simulink model "carPlant_smoothUp_followerStopper_10"  (R2018b)
settings: Solver=VariableStepAuto  StartTime=0.0  StopTime=inf  RelTol=1e-3
undefined symbols (not defined in the file or in its folder): Angular, Linear
libraries: robotlib x13, autolibshared x10, vehdynlibsteering x10
(part 1 of 2)
settings Model: Creator=ckreienk  LastModifiedBy=ckreienk

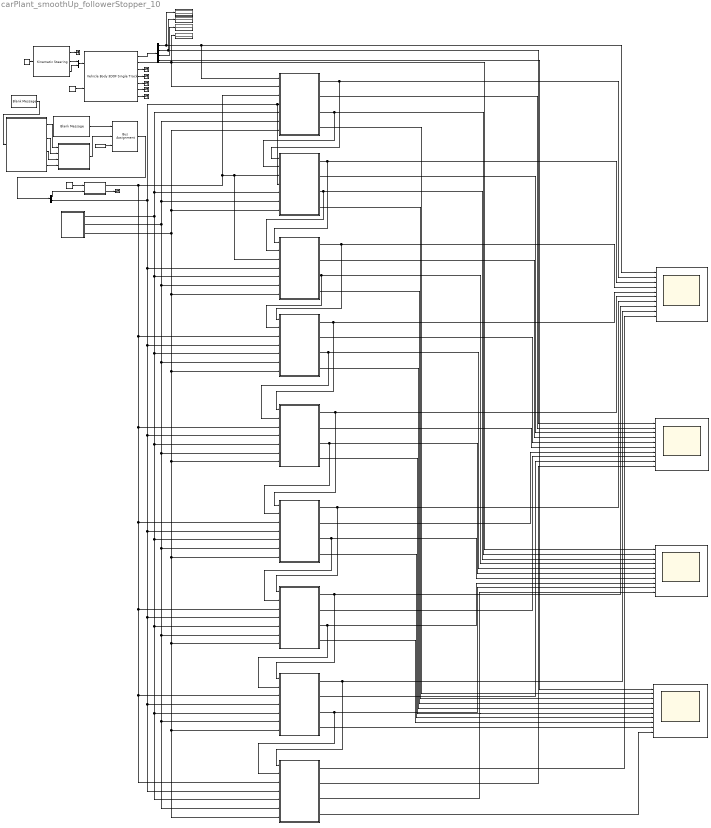
== system carPlant_smoothUp_followerStopper_10 ==
  Acceleration : Scope  NumInputPorts=10
  Blank Message : robotlib/Blank Message  messageClass=Message  entityType=geometry_msgs/Point  messageType=geometry_msgs/Point  SampleTime=inf
      settings: SourceProductBaseCode=RO
  Blank Message Leader : robotlib/Blank Message  messageClass=Message  entityType=geometry_msgs/Twist  messageType=geometry_msgs/Twist  SampleTime=inf
      settings: SourceProductBaseCode=RO
  Bus Assignment7 : BusAssignment  AssignedSignals=Linear.X,Angular.Z
  Bus Selector : BusSelector  OutputSignals=Linear.X,Angular.Z
  Bus Selector2 : BusSelector  OutputSignals=InertFrm.Geom.Disp.X,InertFrm.Geom.Disp.Y,InertFrm.Geom.Disp.Z,BdyFrm.Cg.Acc.xddot
  Constant12 : Constant
  Constant3 : Constant  Value=0
  Dead Man's Switch : Subsystem  TreatAsAtomicUnit=on  mask{stepSize=0.05, timeout=0.2}
      mask prompts: stepSize "Simulation step size"; timeout "Timeout (in seconds)"
      mask help: Interprets whether a new message has been recently received, and if so permits the data in 'value' to be passed through. Otherwise, 0 is outputted from 'safeValue'
      mask Help: Interprets whether a new message has been recently received, and if so permits the data in 'value' to be passed through. Otherwise, 0 is outputted from 'safeValue'
  Display{1..3,7} (4 alike) : Display
  Follower 1 : Subsystem
  Follower 2 : Subsystem
  Follower 3 : Subsystem
  Follower 4 : Subsystem
  Follower 5 : Subsystem
  Follower 6 : Subsystem
  Follower 7 : Subsystem
  Follower 8 : Subsystem
  Follower 9 : Subsystem
  Kinematic Steering : vehdynlibsteering/Kinematic Steering  StrgType=Rack and pinion  StrgRatioType=Constant  Loc=Front  NrmlFctr=0.01  TrckWdth=1  WhlBase=1.524  Db=0  StrgRng=1.25*pi  StrgAngBpts="[-6.2832   -5.0265   -3.7699   -2.5133   -1.2566         0    1.2566    2.5133    3.7699    5.0265    6.2832]"  StrgRatioTbl=|  StrgRatio=100  StrgArmLngth=0.1  RckCsLngth=0.5  TieRodLngth=0.248  D=0.2  PnnRadius=0.0057  PnnRadiusTbl="[0.0055    0.0055    0.0056    0.0057    0.0058    0.0057    0.0057    0.0057    0.0056    0.0055    0.0055]"  RodLngth=0.1  ParaArmLngth=0.9  aMode=2
      | [13.5000   13.3750   13.2500   13.1250   13.0000   13.0000   13.0000   13.1250   13.2500   13.3750   13.5000
      | ]
      settings: SourceProductName=Vehicle Dynamics Blockset
  Lead Vehicle : autolibshared/Vehicle Body 3DOF Single Track  trackMode=Dual  inputMode=External longitudinal velocity  frontSteerMode=on  rearSteerMode=off  windMode=off  muMode=off  extFMode=off  extMMode=off  aMode=2  NF=2  NR=2  m=2000  a=1.4  b=1.6  h=0.35  X_o=45  xdot_o=0  CalphaMode=off  sigmaMode=on  d=0  w=[1.4,1.4]  Cy_f=12e3  Cy_r=11e3  sigma_f=.1  sigma_r=.1  alpha_f_brk=[-.1 .1]  Cy_f_data=[-9e3 9e3]  alpha_r_brk=[-.1 .1]  Cy_r_data=[-9e3 9e3]  Y_o=0  ydot_o=0  Izz=4000  psi_o=0  r_o=0  Af=2  Cd=.3  Cl=.1  Cpm=.1  beta_w=[0:0.01:0.3]  Cs=[0:0.03:0.9]  Cym=[0:0.01:0.3]  Pabs=101325  Tair=273  g=9.81  mu=1  xdot_tol=.01  Fznom=5000  Fxtire_sat=7e4  Fytire_sat=7e4  longOff=0  latOff=0  vertOff=0
      settings: SourceProductName=Powertrain Blockset  SourceProductBaseCode=PW
  MATLAB Function : MATLAB Function  TreatAsAtomicUnit=on
  Parameters : Subsystem
  Random Number : RandomNumber  Mean=3  Variance=3  SampleTime=0.1
  Steering angle : Constant  Value=0.0
  Terminator{5..10,15} (7 alike) : Terminator
  Vector Concatenate : Concatenate
  Velocity : Scope  NumInputPorts=10
  X-Position : Scope  NumInputPorts=10
  Y-Position : Scope  NumInputPorts=10
  smoothUp Parameters : Subsystem
  wires:
  Lead Vehicle/6 -> Terminator9/1
  Bus Selector2/3 -> Display3/1  "<Z>"
  smoothUp Parameters/1(max_speed) -> MATLAB Function/1(max_speed)
  Bus Selector/1 -> Dead Man's Switch/2(value)  "<X>"
  Blank Message Leader/1 -> Bus Assignment7/1
  MATLAB Function/1(u_out) -> Bus Assignment7/2
  Bus Selector2/4 -> Acceleration/1  "<xddot>"
  Lead Vehicle/4 -> Terminator7/1
  Lead Vehicle/2 -> Display7/1, Velocity/1, Follower 1/2(V_(n-1))
  Lead Vehicle/3 -> Terminator6/1
  Lead Vehicle/1 -> Bus Selector2/1
  Dead Man's Switch/2(timedOut) -> Terminator15/1
  Blank Message/1 -> smoothUp Parameters/1(In1)
  Bus Selector2/2 -> Y-Position/1, Display2/1  "<Y>"
  Constant3/1 -> Kinematic Steering/1
  Lead Vehicle/7 -> Terminator10/1
  Kinematic Steering/3 -> Vector Concatenate/2
  Bus Selector2/1 -> Display1/1, X-Position/1, Follower 1/1(X_(n-1))  "<X>"
  Lead Vehicle/5 -> Terminator8/1
  Bus Assignment7/1 -> Bus Selector/1
  Kinematic Steering/1 -> Terminator5/1
  Kinematic Steering/2 -> Vector Concatenate/1
  Random Number/1 -> Lead Vehicle/2
  Constant12/1 -> Dead Man's Switch/1(IsNew)
  Steering angle/1 -> Bus Assignment7/3
  Vector Concatenate/1 -> Lead Vehicle/1
  Dead Man's Switch/1(safeValue) -> Follower 9/3(reference velocity), Follower 8/3(reference velocity), Follower 7/3(reference velocity), Follower 6/3(reference velocity), Follower 5/3(reference velocity), Follower 4/3(reference velocity), Follower 3/3(reference velocity), Follower 2/3(reference velocity), Follower 1/3(reference velocity)
  Bus Selector/2 -> Follower 9/4(reference angle), Follower 8/4(reference angle), Follower 7/4(reference angle), Follower 6/4(reference angle), Follower 5/4(reference angle), Follower 4/4(reference angle), Follower 3/4(reference angle), Follower 2/4(reference angle), Follower 1/4(reference angle)  "<Z>"
  Parameters/1(alpha) -> Follower 9/5(alpha), Follower 8/5(alpha), Follower 7/5(alpha), Follower 6/5(alpha), Follower 5/5(alpha), Follower 4/5(alpha), Follower 3/5(alpha), Follower 2/5(alpha), Follower 1/5(alpha)
  Parameters/2(omega_1) -> Follower 9/6(omega1), Follower 8/6(omega1), Follower 7/6(omega1), Follower 6/6(omega1), Follower 5/6(omega1), Follower 4/6(omega1), Follower 3/6(omega1), Follower 2/6(omega1), Follower 1/6(omega1)
  Parameters/3(omega_3) -> Follower 9/7(omega3), Follower 8/7(omega3), Follower 7/7(omega3), Follower 6/7(omega3), Follower 5/7(omega3), Follower 4/7(omega3), Follower 3/7(omega3), Follower 2/7(omega3), Follower 1/7(omega3)
  Follower 1/1(X_n) -> Follower 2/1(X_(n-1)), X-Position/2
  Follower 1/2(Y_n) -> Y-Position/2
  Follower 1/3(V_n) -> Follower 2/2(V_(n-1)), Velocity/2
  Follower 1/4(A_n) -> Acceleration/2
  Follower 2/1(X_n) -> Follower 3/1(X_(n-1)), X-Position/3
  Follower 2/3(V_n) -> Follower 3/2(V_(n-1)), Velocity/3
  Follower 3/1(X_n) -> Follower 4/1(X_(n-1)), X-Position/4
  Follower 3/3(V_n) -> Follower 4/2(V_(n-1)), Velocity/4
  Follower 4/1(X_n) -> X-Position/5, Follower 5/1(X_(n-1))
  Follower 4/3(V_n) -> Follower 5/2(V_(n-1)), Velocity/5
  Follower 5/3(V_n) -> Follower 6/2(V_(n-1)), Velocity/6
  Follower 5/1(X_n) -> X-Position/6, Follower 6/1(X_(n-1))
  Follower 6/1(X_n) -> X-Position/7, Follower 7/1(X_(n-1))
  Follower 6/3(V_n) -> Follower 7/2(V_(n-1)), Velocity/7
  Follower 7/1(X_n) -> X-Position/8, Follower 8/1(X_(n-1))
  Follower 7/3(V_n) -> Velocity/8, Follower 8/2(V_(n-1))
  Follower 8/1(X_n) -> X-Position/9, Follower 9/1(X_(n-1))
  Follower 8/3(V_n) -> Velocity/9, Follower 9/2(V_(n-1))
  Follower 9/1(X_n) -> X-Position/10
  Follower 2/2(Y_n) -> Y-Position/3
  Follower 3/2(Y_n) -> Y-Position/4
  Follower 4/2(Y_n) -> Y-Position/5
  Follower 5/2(Y_n) -> Y-Position/6
  Follower 6/2(Y_n) -> Y-Position/7
  Follower 7/2(Y_n) -> Y-Position/8
  Follower 8/2(Y_n) -> Y-Position/9
  Follower 9/2(Y_n) -> Y-Position/10
  Follower 9/3(V_n) -> Velocity/10
  Follower 2/4(A_n) -> Acceleration/3
  Follower 3/4(A_n) -> Acceleration/4
  Follower 4/4(A_n) -> Acceleration/5
  Follower 5/4(A_n) -> Acceleration/6
  Follower 6/4(A_n) -> Acceleration/7
  Follower 7/4(A_n) -> Acceleration/8
  Follower 8/4(A_n) -> Acceleration/9
  Follower 9/4(A_n) -> Acceleration/10
  smoothUp Parameters/2(reference_vel) -> MATLAB Function/2(vel)
  smoothUp Parameters/3(max_accel) -> MATLAB Function/3(max_accel)
  smoothUp Parameters/4(max_decel) -> MATLAB Function/4(max_decel)

== system carPlant_smoothUp_followerStopper_10/Dead Man's Switch ==
  note: The timeout value, and step size, are critical to set correctly here.
  IsNew : Inport
  value : Inport  Port=2
  Simulate step size : Constant  Value=stepSize
  Timeout in seconds : Constant  Value=timeout
  timeout set to 0 output : MATLAB Function  TreatAsAtomicUnit=on
  safeValue : Outport  InitialOutput=[0]
  timedOut : Outport  Port=2  InitialOutput=[0]
  wires:
  Simulate step size/1 -> timeout set to 0 output/4(stepSize)
  timeout set to 0 output/2(timedOut) -> timedOut/1
  Timeout in seconds/1 -> timeout set to 0 output/3(timeout)
  value/1 -> timeout set to 0 output/2(value)
  timeout set to 0 output/1(safeValue) -> safeValue/1
  IsNew/1 -> timeout set to 0 output/1(isNew)

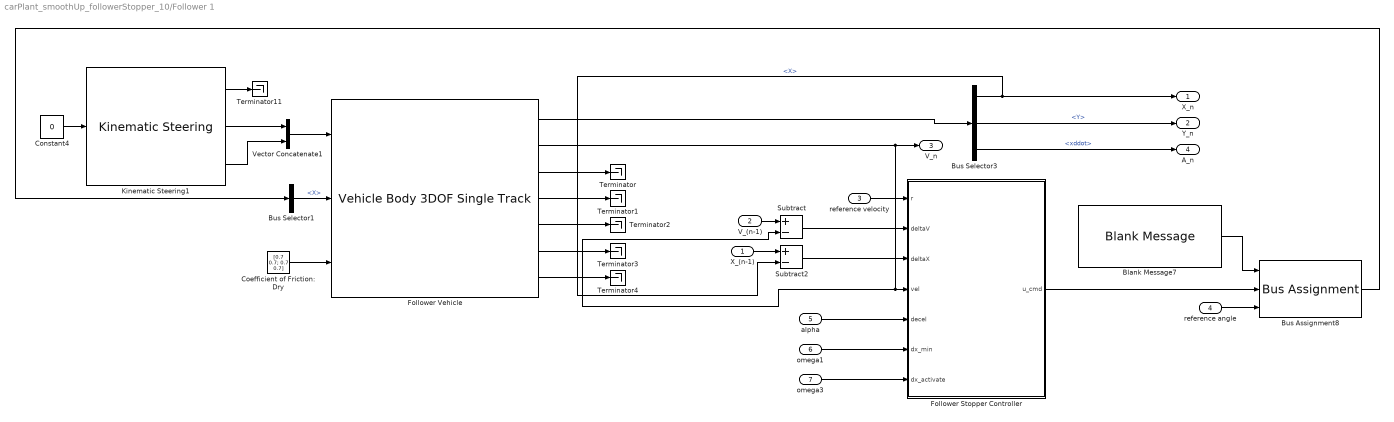
== system carPlant_smoothUp_followerStopper_10/Follower 1 ==
  X_(n-1) : Inport
  V_(n-1) : Inport  Port=2
  reference velocity : Inport  Port=3
  reference angle : Inport  Port=4
  alpha : Inport  Port=5
  omega1 : Inport  Port=6
  omega3 : Inport  Port=7
  Blank Message7 : robotlib/Blank Message  messageClass=Message  entityType=geometry_msgs/Twist  messageType=geometry_msgs/Twist  SampleTime=inf
      settings: SourceProductBaseCode=RO
  Bus Assignment8 : BusAssignment  AssignedSignals=Linear.X,Angular.Z
  Bus Selector1 : BusSelector  OutputSignals=Linear.X
  Bus Selector3 : BusSelector  OutputSignals=InertFrm.Geom.Disp.X,InertFrm.Geom.Disp.Y,BdyFrm.Cg.Acc.xddot
  Coefficient of Friction: Dry : Constant  Value=[0.7 0.7; 0.7 0.7]
  Constant4 : Constant  Value=0
  Follower Stopper Controller : Subsystem
  Follower Vehicle : autolibshared/Vehicle Body 3DOF Single Track  trackMode=Dual  inputMode=External longitudinal velocity  frontSteerMode=on  rearSteerMode=off  windMode=off  muMode=on  extFMode=off  extMMode=off  aMode=2  NF=2  NR=2  m=2000  a=1.4  b=1.6  h=0.35  X_o=40  xdot_o=0  CalphaMode=off  sigmaMode=on  d=0  w=[1.4,1.4]  Cy_f=12e3  Cy_r=11e3  sigma_f=.1  sigma_r=.1  alpha_f_brk=[-.1 .1]  Cy_f_data=[-9e3 9e3]  alpha_r_brk=[-.1 .1]  Cy_r_data=[-9e3 9e3]  Y_o=0  ydot_o=0  Izz=4000  psi_o=0  r_o=0  Af=2  Cd=.3  Cl=.1  Cpm=.1  beta_w=[0:0.01:0.3]  Cs=[0:0.03:0.9]  Cym=[0:0.01:0.3]  Pabs=101325  Tair=273  g=9.81  mu=1  xdot_tol=.01  Fznom=5000  Fxtire_sat=7e4  Fytire_sat=7e4  longOff=0  latOff=0  vertOff=0
      settings: SourceProductName=Powertrain Blockset  SourceProductBaseCode=PW
  Kinematic Steering1 : vehdynlibsteering/Kinematic Steering  StrgType=Rack and pinion  StrgRatioType=Constant  Loc=Front  NrmlFctr=0.01  TrckWdth=1  WhlBase=1.524  Db=0  StrgRng=1.25*pi  StrgAngBpts="[-6.2832   -5.0265   -3.7699   -2.5133   -1.2566         0    1.2566    2.5133    3.7699    5.0265    6.2832]"  StrgRatioTbl=|  StrgRatio=100  StrgArmLngth=0.1  RckCsLngth=0.5  TieRodLngth=0.248  D=0.2  PnnRadius=0.0057  PnnRadiusTbl="[0.0055    0.0055    0.0056    0.0057    0.0058    0.0057    0.0057    0.0057    0.0056    0.0055    0.0055]"  RodLngth=0.1  ParaArmLngth=0.9  aMode=2
      | [13.5000   13.3750   13.2500   13.1250   13.0000   13.0000   13.0000   13.1250   13.2500   13.3750   13.5000
      | ]
      settings: SourceProductName=Vehicle Dynamics Blockset
  Subtract : Sum  Inputs=+-
  Subtract2 : Sum  Inputs=+-
  Terminator{,1..4,11} (6 alike) : Terminator
  Vector Concatenate1 : Concatenate
  X_n : Outport
  Y_n : Outport  Port=2
  V_n : Outport  Port=3
  A_n : Outport  Port=4
  wires:
  Constant4/1 -> Kinematic Steering1/1
  Bus Assignment8/1 -> Bus Selector1/1
  Follower Vehicle/4 -> Terminator1/1
  V_(n-1)/1 -> Subtract/1
  Kinematic Steering1/1 -> Terminator11/1
  Bus Selector3/1 -> Subtract2/2, X_n/1  "<X>"
  alpha/1 -> Follower Stopper Controller/5(decel)
  omega1/1 -> Follower Stopper Controller/6(dx_min)
  Coefficient of Friction: Dry/1 -> Follower Vehicle/3
  Follower Vehicle/7 -> Terminator4/1
  Subtract2/1 -> Follower Stopper Controller/3(deltaX)
  Vector Concatenate1/1 -> Follower Vehicle/1
  X_(n-1)/1 -> Subtract2/1
  omega3/1 -> Follower Stopper Controller/7(dx_activate)
  Bus Selector3/3 -> A_n/1  "<xddot>"
  Bus Selector3/2 -> Y_n/1  "<Y>"
  reference velocity/1 -> Follower Stopper Controller/1(r)
  Follower Vehicle/2 -> V_n/1, Subtract/2, Follower Stopper Controller/4(vel)
  Follower Vehicle/1 -> Bus Selector3/1
  Subtract/1 -> Follower Stopper Controller/2(deltaV)
  Follower Vehicle/5 -> Terminator2/1
  Follower Stopper Controller/1(u_cmd) -> Bus Assignment8/2
  Blank Message7/1 -> Bus Assignment8/1
  Bus Selector1/1 -> Follower Vehicle/2  "<X>"
  Kinematic Steering1/3 -> Vector Concatenate1/2
  Kinematic Steering1/2 -> Vector Concatenate1/1
  reference angle/1 -> Bus Assignment8/3
  Follower Vehicle/6 -> Terminator3/1
  Follower Vehicle/3 -> Terminator/1

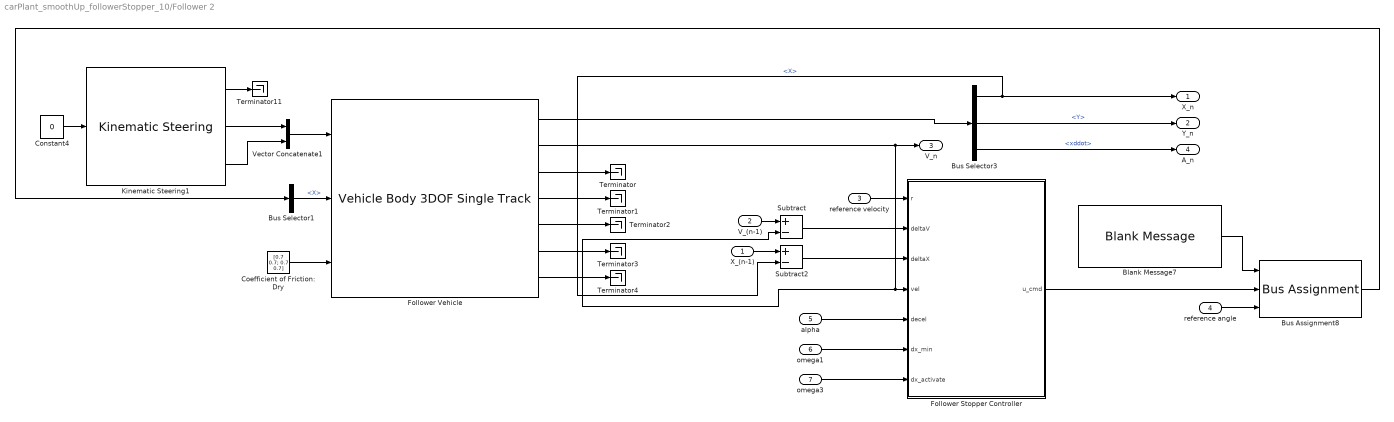
== system carPlant_smoothUp_followerStopper_10/Follower 2 ==
  X_(n-1) : Inport
  V_(n-1) : Inport  Port=2
  reference velocity : Inport  Port=3
  reference angle : Inport  Port=4
  alpha : Inport  Port=5
  omega1 : Inport  Port=6
  omega3 : Inport  Port=7
  Blank Message7 : robotlib/Blank Message  messageClass=Message  entityType=geometry_msgs/Twist  messageType=geometry_msgs/Twist  SampleTime=inf
      settings: SourceProductBaseCode=RO
  Bus Assignment8 : BusAssignment  AssignedSignals=Linear.X,Angular.Z
  Bus Selector1 : BusSelector  OutputSignals=Linear.X
  Bus Selector3 : BusSelector  OutputSignals=InertFrm.Geom.Disp.X,InertFrm.Geom.Disp.Y,BdyFrm.Cg.Acc.xddot
  Coefficient of Friction: Dry : Constant  Value=[0.7 0.7; 0.7 0.7]
  Constant4 : Constant  Value=0
  Follower Stopper Controller : Subsystem
  Follower Vehicle : autolibshared/Vehicle Body 3DOF Single Track  trackMode=Dual  inputMode=External longitudinal velocity  frontSteerMode=on  rearSteerMode=off  windMode=off  muMode=on  extFMode=off  extMMode=off  aMode=2  NF=2  NR=2  m=2000  a=1.4  b=1.6  h=0.35  X_o=35  xdot_o=0  CalphaMode=off  sigmaMode=on  d=0  w=[1.4,1.4]  Cy_f=12e3  Cy_r=11e3  sigma_f=.1  sigma_r=.1  alpha_f_brk=[-.1 .1]  Cy_f_data=[-9e3 9e3]  alpha_r_brk=[-.1 .1]  Cy_r_data=[-9e3 9e3]  Y_o=0  ydot_o=0  Izz=4000  psi_o=0  r_o=0  Af=2  Cd=.3  Cl=.1  Cpm=.1  beta_w=[0:0.01:0.3]  Cs=[0:0.03:0.9]  Cym=[0:0.01:0.3]  Pabs=101325  Tair=273  g=9.81  mu=1  xdot_tol=.01  Fznom=5000  Fxtire_sat=7e4  Fytire_sat=7e4  longOff=0  latOff=0  vertOff=0
      settings: SourceProductName=Powertrain Blockset  SourceProductBaseCode=PW
  Kinematic Steering1 : vehdynlibsteering/Kinematic Steering  StrgType=Rack and pinion  StrgRatioType=Constant  Loc=Front  NrmlFctr=0.01  TrckWdth=1  WhlBase=1.524  Db=0  StrgRng=1.25*pi  StrgAngBpts="[-6.2832   -5.0265   -3.7699   -2.5133   -1.2566         0    1.2566    2.5133    3.7699    5.0265    6.2832]"  StrgRatioTbl=|  StrgRatio=100  StrgArmLngth=0.1  RckCsLngth=0.5  TieRodLngth=0.248  D=0.2  PnnRadius=0.0057  PnnRadiusTbl="[0.0055    0.0055    0.0056    0.0057    0.0058    0.0057    0.0057    0.0057    0.0056    0.0055    0.0055]"  RodLngth=0.1  ParaArmLngth=0.9  aMode=2
      | [13.5000   13.3750   13.2500   13.1250   13.0000   13.0000   13.0000   13.1250   13.2500   13.3750   13.5000
      | ]
      settings: SourceProductName=Vehicle Dynamics Blockset
  Subtract : Sum  Inputs=+-
  Subtract2 : Sum  Inputs=+-
  Terminator{,1..4,11} (6 alike) : Terminator
  Vector Concatenate1 : Concatenate
  X_n : Outport
  Y_n : Outport  Port=2
  V_n : Outport  Port=3
  A_n : Outport  Port=4
  wires:
  Follower Vehicle/3 -> Terminator/1
  Follower Vehicle/6 -> Terminator3/1
  reference angle/1 -> Bus Assignment8/3
  Kinematic Steering1/2 -> Vector Concatenate1/1
  Kinematic Steering1/3 -> Vector Concatenate1/2
  Bus Selector1/1 -> Follower Vehicle/2  "<X>"
  Blank Message7/1 -> Bus Assignment8/1
  Follower Stopper Controller/1(u_cmd) -> Bus Assignment8/2
  Follower Vehicle/5 -> Terminator2/1
  Subtract/1 -> Follower Stopper Controller/2(deltaV)
  Follower Vehicle/1 -> Bus Selector3/1
  Follower Vehicle/2 -> Follower Stopper Controller/4(vel), Subtract/2, V_n/1
  reference velocity/1 -> Follower Stopper Controller/1(r)
  Bus Selector3/2 -> Y_n/1  "<Y>"
  Bus Selector3/3 -> A_n/1  "<xddot>"
  omega3/1 -> Follower Stopper Controller/7(dx_activate)
  X_(n-1)/1 -> Subtract2/1
  Vector Concatenate1/1 -> Follower Vehicle/1
  Subtract2/1 -> Follower Stopper Controller/3(deltaX)
  Follower Vehicle/7 -> Terminator4/1
  Coefficient of Friction: Dry/1 -> Follower Vehicle/3
  omega1/1 -> Follower Stopper Controller/6(dx_min)
  alpha/1 -> Follower Stopper Controller/5(decel)
  Bus Selector3/1 -> X_n/1, Subtract2/2  "<X>"
  Kinematic Steering1/1 -> Terminator11/1
  V_(n-1)/1 -> Subtract/1
  Follower Vehicle/4 -> Terminator1/1
  Bus Assignment8/1 -> Bus Selector1/1
  Constant4/1 -> Kinematic Steering1/1

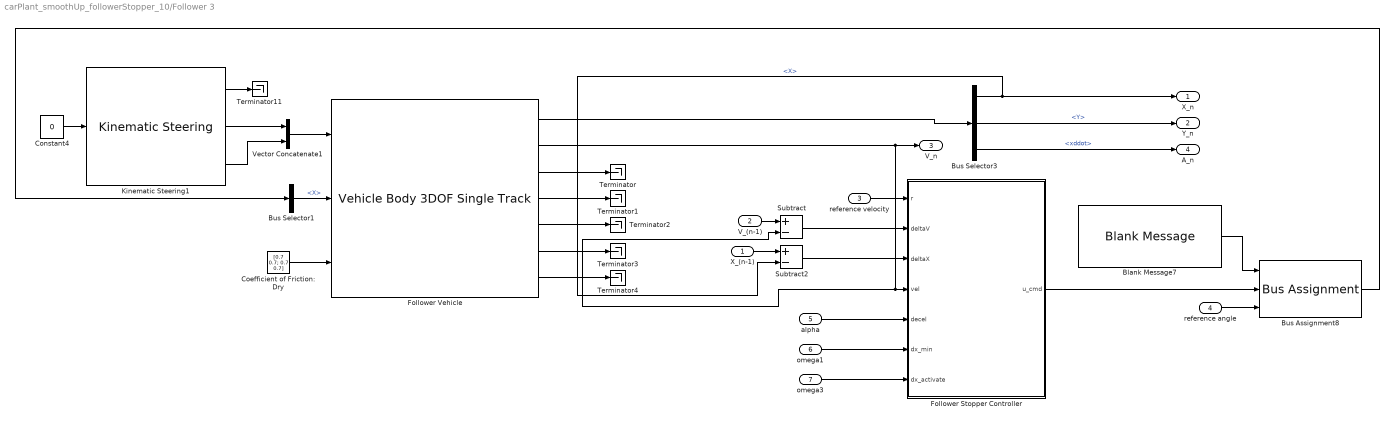
== system carPlant_smoothUp_followerStopper_10/Follower 3 ==
  X_(n-1) : Inport
  V_(n-1) : Inport  Port=2
  reference velocity : Inport  Port=3
  reference angle : Inport  Port=4
  alpha : Inport  Port=5
  omega1 : Inport  Port=6
  omega3 : Inport  Port=7
  Blank Message7 : robotlib/Blank Message  messageClass=Message  entityType=geometry_msgs/Twist  messageType=geometry_msgs/Twist  SampleTime=inf
      settings: SourceProductBaseCode=RO
  Bus Assignment8 : BusAssignment  AssignedSignals=Linear.X,Angular.Z
  Bus Selector1 : BusSelector  OutputSignals=Linear.X
  Bus Selector3 : BusSelector  OutputSignals=InertFrm.Geom.Disp.X,InertFrm.Geom.Disp.Y,BdyFrm.Cg.Acc.xddot
  Coefficient of Friction: Dry : Constant  Value=[0.7 0.7; 0.7 0.7]
  Constant4 : Constant  Value=0
  Follower Stopper Controller : Subsystem
  Follower Vehicle : autolibshared/Vehicle Body 3DOF Single Track  trackMode=Dual  inputMode=External longitudinal velocity  frontSteerMode=on  rearSteerMode=off  windMode=off  muMode=on  extFMode=off  extMMode=off  aMode=2  NF=2  NR=2  m=2000  a=1.4  b=1.6  h=0.35  X_o=30  xdot_o=0  CalphaMode=off  sigmaMode=on  d=0  w=[1.4,1.4]  Cy_f=12e3  Cy_r=11e3  sigma_f=.1  sigma_r=.1  alpha_f_brk=[-.1 .1]  Cy_f_data=[-9e3 9e3]  alpha_r_brk=[-.1 .1]  Cy_r_data=[-9e3 9e3]  Y_o=0  ydot_o=0  Izz=4000  psi_o=0  r_o=0  Af=2  Cd=.3  Cl=.1  Cpm=.1  beta_w=[0:0.01:0.3]  Cs=[0:0.03:0.9]  Cym=[0:0.01:0.3]  Pabs=101325  Tair=273  g=9.81  mu=1  xdot_tol=.01  Fznom=5000  Fxtire_sat=7e4  Fytire_sat=7e4  longOff=0  latOff=0  vertOff=0
      settings: SourceProductName=Powertrain Blockset  SourceProductBaseCode=PW
  Kinematic Steering1 : vehdynlibsteering/Kinematic Steering  StrgType=Rack and pinion  StrgRatioType=Constant  Loc=Front  NrmlFctr=0.01  TrckWdth=1  WhlBase=1.524  Db=0  StrgRng=1.25*pi  StrgAngBpts="[-6.2832   -5.0265   -3.7699   -2.5133   -1.2566         0    1.2566    2.5133    3.7699    5.0265    6.2832]"  StrgRatioTbl=|  StrgRatio=100  StrgArmLngth=0.1  RckCsLngth=0.5  TieRodLngth=0.248  D=0.2  PnnRadius=0.0057  PnnRadiusTbl="[0.0055    0.0055    0.0056    0.0057    0.0058    0.0057    0.0057    0.0057    0.0056    0.0055    0.0055]"  RodLngth=0.1  ParaArmLngth=0.9  aMode=2
      | [13.5000   13.3750   13.2500   13.1250   13.0000   13.0000   13.0000   13.1250   13.2500   13.3750   13.5000
      | ]
      settings: SourceProductName=Vehicle Dynamics Blockset
  Subtract : Sum  Inputs=+-
  Subtract2 : Sum  Inputs=+-
  Terminator{,1..4,11} (6 alike) : Terminator
  Vector Concatenate1 : Concatenate
  X_n : Outport
  Y_n : Outport  Port=2
  V_n : Outport  Port=3
  A_n : Outport  Port=4
  wires:
  Constant4/1 -> Kinematic Steering1/1
  Bus Assignment8/1 -> Bus Selector1/1
  Follower Vehicle/4 -> Terminator1/1
  V_(n-1)/1 -> Subtract/1
  Kinematic Steering1/1 -> Terminator11/1
  Bus Selector3/1 -> Subtract2/2, X_n/1  "<X>"
  alpha/1 -> Follower Stopper Controller/5(decel)
  omega1/1 -> Follower Stopper Controller/6(dx_min)
  Coefficient of Friction: Dry/1 -> Follower Vehicle/3
  Follower Vehicle/7 -> Terminator4/1
  Subtract2/1 -> Follower Stopper Controller/3(deltaX)
  Vector Concatenate1/1 -> Follower Vehicle/1
  X_(n-1)/1 -> Subtract2/1
  omega3/1 -> Follower Stopper Controller/7(dx_activate)
  Bus Selector3/3 -> A_n/1  "<xddot>"
  Bus Selector3/2 -> Y_n/1  "<Y>"
  reference velocity/1 -> Follower Stopper Controller/1(r)
  Follower Vehicle/2 -> V_n/1, Subtract/2, Follower Stopper Controller/4(vel)
  Follower Vehicle/1 -> Bus Selector3/1
  Subtract/1 -> Follower Stopper Controller/2(deltaV)
  Follower Vehicle/5 -> Terminator2/1
  Follower Stopper Controller/1(u_cmd) -> Bus Assignment8/2
  Blank Message7/1 -> Bus Assignment8/1
  Bus Selector1/1 -> Follower Vehicle/2  "<X>"
  Kinematic Steering1/3 -> Vector Concatenate1/2
  Kinematic Steering1/2 -> Vector Concatenate1/1
  reference angle/1 -> Bus Assignment8/3
  Follower Vehicle/6 -> Terminator3/1
  Follower Vehicle/3 -> Terminator/1

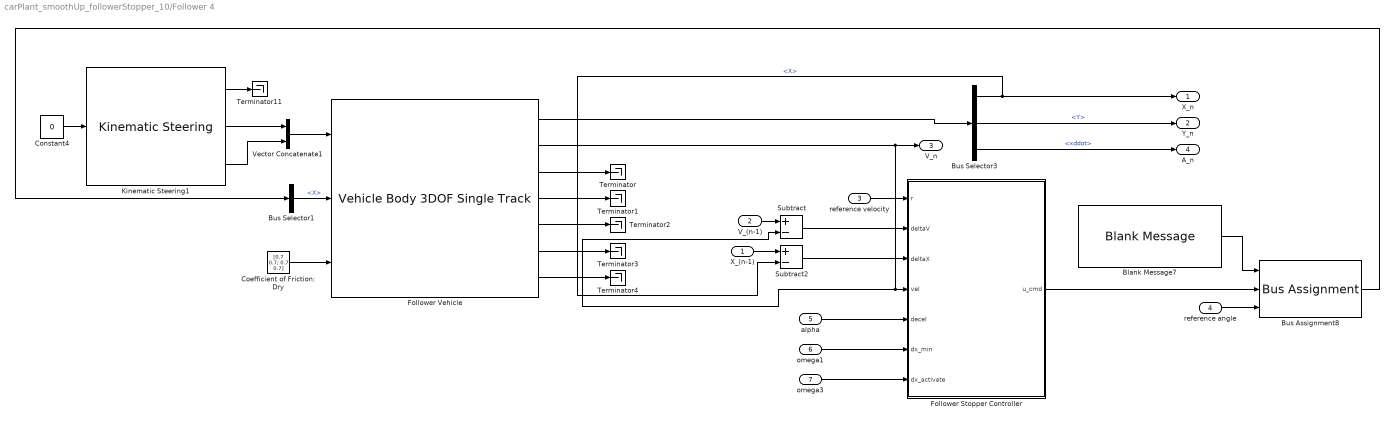
== system carPlant_smoothUp_followerStopper_10/Follower 4 ==
  X_(n-1) : Inport
  V_(n-1) : Inport  Port=2
  reference velocity : Inport  Port=3
  reference angle : Inport  Port=4
  alpha : Inport  Port=5
  omega1 : Inport  Port=6
  omega3 : Inport  Port=7
  Blank Message7 : robotlib/Blank Message  messageClass=Message  entityType=geometry_msgs/Twist  messageType=geometry_msgs/Twist  SampleTime=inf
      settings: SourceProductBaseCode=RO
  Bus Assignment8 : BusAssignment  AssignedSignals=Linear.X,Angular.Z
  Bus Selector1 : BusSelector  OutputSignals=Linear.X
  Bus Selector3 : BusSelector  OutputSignals=InertFrm.Geom.Disp.X,InertFrm.Geom.Disp.Y,BdyFrm.Cg.Acc.xddot
  Coefficient of Friction: Dry : Constant  Value=[0.7 0.7; 0.7 0.7]
  Constant4 : Constant  Value=0
  Follower Stopper Controller : Subsystem
  Follower Vehicle : autolibshared/Vehicle Body 3DOF Single Track  trackMode=Dual  inputMode=External longitudinal velocity  frontSteerMode=on  rearSteerMode=off  windMode=off  muMode=on  extFMode=off  extMMode=off  aMode=2  NF=2  NR=2  m=2000  a=1.4  b=1.6  h=0.35  X_o=25  xdot_o=0  CalphaMode=off  sigmaMode=on  d=0  w=[1.4,1.4]  Cy_f=12e3  Cy_r=11e3  sigma_f=.1  sigma_r=.1  alpha_f_brk=[-.1 .1]  Cy_f_data=[-9e3 9e3]  alpha_r_brk=[-.1 .1]  Cy_r_data=[-9e3 9e3]  Y_o=0  ydot_o=0  Izz=4000  psi_o=0  r_o=0  Af=2  Cd=.3  Cl=.1  Cpm=.1  beta_w=[0:0.01:0.3]  Cs=[0:0.03:0.9]  Cym=[0:0.01:0.3]  Pabs=101325  Tair=273  g=9.81  mu=1  xdot_tol=.01  Fznom=5000  Fxtire_sat=7e4  Fytire_sat=7e4  longOff=0  latOff=0  vertOff=0
      settings: SourceProductName=Powertrain Blockset  SourceProductBaseCode=PW
  Kinematic Steering1 : vehdynlibsteering/Kinematic Steering  StrgType=Rack and pinion  StrgRatioType=Constant  Loc=Front  NrmlFctr=0.01  TrckWdth=1  WhlBase=1.524  Db=0  StrgRng=1.25*pi  StrgAngBpts="[-6.2832   -5.0265   -3.7699   -2.5133   -1.2566         0    1.2566    2.5133    3.7699    5.0265    6.2832]"  StrgRatioTbl=|  StrgRatio=100  StrgArmLngth=0.1  RckCsLngth=0.5  TieRodLngth=0.248  D=0.2  PnnRadius=0.0057  PnnRadiusTbl="[0.0055    0.0055    0.0056    0.0057    0.0058    0.0057    0.0057    0.0057    0.0056    0.0055    0.0055]"  RodLngth=0.1  ParaArmLngth=0.9  aMode=2
      | [13.5000   13.3750   13.2500   13.1250   13.0000   13.0000   13.0000   13.1250   13.2500   13.3750   13.5000
      | ]
      settings: SourceProductName=Vehicle Dynamics Blockset
  Subtract : Sum  Inputs=+-
  Subtract2 : Sum  Inputs=+-
  Terminator{,1..4,11} (6 alike) : Terminator
  Vector Concatenate1 : Concatenate
  X_n : Outport
  Y_n : Outport  Port=2
  V_n : Outport  Port=3
  A_n : Outport  Port=4
  wires:
  Follower Vehicle/3 -> Terminator/1
  Follower Vehicle/6 -> Terminator3/1
  reference angle/1 -> Bus Assignment8/3
  Kinematic Steering1/2 -> Vector Concatenate1/1
  Kinematic Steering1/3 -> Vector Concatenate1/2
  Bus Selector1/1 -> Follower Vehicle/2  "<X>"
  Blank Message7/1 -> Bus Assignment8/1
  Follower Stopper Controller/1(u_cmd) -> Bus Assignment8/2
  Follower Vehicle/5 -> Terminator2/1
  Subtract/1 -> Follower Stopper Controller/2(deltaV)
  Follower Vehicle/1 -> Bus Selector3/1
  Follower Vehicle/2 -> Follower Stopper Controller/4(vel), Subtract/2, V_n/1
  reference velocity/1 -> Follower Stopper Controller/1(r)
  Bus Selector3/2 -> Y_n/1  "<Y>"
  Bus Selector3/3 -> A_n/1  "<xddot>"
  omega3/1 -> Follower Stopper Controller/7(dx_activate)
  X_(n-1)/1 -> Subtract2/1
  Vector Concatenate1/1 -> Follower Vehicle/1
  Subtract2/1 -> Follower Stopper Controller/3(deltaX)
  Follower Vehicle/7 -> Terminator4/1
  Coefficient of Friction: Dry/1 -> Follower Vehicle/3
  omega1/1 -> Follower Stopper Controller/6(dx_min)
  alpha/1 -> Follower Stopper Controller/5(decel)
  Bus Selector3/1 -> X_n/1, Subtract2/2  "<X>"
  Kinematic Steering1/1 -> Terminator11/1
  V_(n-1)/1 -> Subtract/1
  Follower Vehicle/4 -> Terminator1/1
  Bus Assignment8/1 -> Bus Selector1/1
  Constant4/1 -> Kinematic Steering1/1

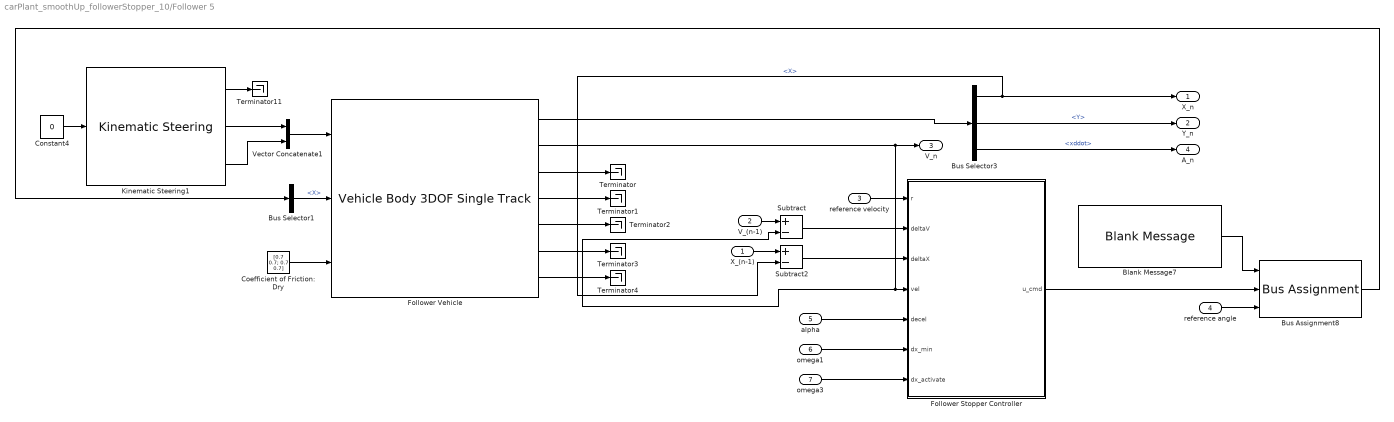
== system carPlant_smoothUp_followerStopper_10/Follower 5 ==
  X_(n-1) : Inport
  V_(n-1) : Inport  Port=2
  reference velocity : Inport  Port=3
  reference angle : Inport  Port=4
  alpha : Inport  Port=5
  omega1 : Inport  Port=6
  omega3 : Inport  Port=7
  Blank Message7 : robotlib/Blank Message  messageClass=Message  entityType=geometry_msgs/Twist  messageType=geometry_msgs/Twist  SampleTime=inf
      settings: SourceProductBaseCode=RO
  Bus Assignment8 : BusAssignment  AssignedSignals=Linear.X,Angular.Z
  Bus Selector1 : BusSelector  OutputSignals=Linear.X
  Bus Selector3 : BusSelector  OutputSignals=InertFrm.Geom.Disp.X,InertFrm.Geom.Disp.Y,BdyFrm.Cg.Acc.xddot
  Coefficient of Friction: Dry : Constant  Value=[0.7 0.7; 0.7 0.7]
  Constant4 : Constant  Value=0
  Follower Stopper Controller : Subsystem
  Follower Vehicle : autolibshared/Vehicle Body 3DOF Single Track  trackMode=Dual  inputMode=External longitudinal velocity  frontSteerMode=on  rearSteerMode=off  windMode=off  muMode=on  extFMode=off  extMMode=off  aMode=2  NF=2  NR=2  m=2000  a=1.4  b=1.6  h=0.35  X_o=20  xdot_o=0  CalphaMode=off  sigmaMode=on  d=0  w=[1.4,1.4]  Cy_f=12e3  Cy_r=11e3  sigma_f=.1  sigma_r=.1  alpha_f_brk=[-.1 .1]  Cy_f_data=[-9e3 9e3]  alpha_r_brk=[-.1 .1]  Cy_r_data=[-9e3 9e3]  Y_o=0  ydot_o=0  Izz=4000  psi_o=0  r_o=0  Af=2  Cd=.3  Cl=.1  Cpm=.1  beta_w=[0:0.01:0.3]  Cs=[0:0.03:0.9]  Cym=[0:0.01:0.3]  Pabs=101325  Tair=273  g=9.81  mu=1  xdot_tol=.01  Fznom=5000  Fxtire_sat=7e4  Fytire_sat=7e4  longOff=0  latOff=0  vertOff=0
      settings: SourceProductName=Powertrain Blockset  SourceProductBaseCode=PW
  Kinematic Steering1 : vehdynlibsteering/Kinematic Steering  StrgType=Rack and pinion  StrgRatioType=Constant  Loc=Front  NrmlFctr=0.01  TrckWdth=1  WhlBase=1.524  Db=0  StrgRng=1.25*pi  StrgAngBpts="[-6.2832   -5.0265   -3.7699   -2.5133   -1.2566         0    1.2566    2.5133    3.7699    5.0265    6.2832]"  StrgRatioTbl=|  StrgRatio=100  StrgArmLngth=0.1  RckCsLngth=0.5  TieRodLngth=0.248  D=0.2  PnnRadius=0.0057  PnnRadiusTbl="[0.0055    0.0055    0.0056    0.0057    0.0058    0.0057    0.0057    0.0057    0.0056    0.0055    0.0055]"  RodLngth=0.1  ParaArmLngth=0.9  aMode=2
      | [13.5000   13.3750   13.2500   13.1250   13.0000   13.0000   13.0000   13.1250   13.2500   13.3750   13.5000
      | ]
      settings: SourceProductName=Vehicle Dynamics Blockset
  Subtract : Sum  Inputs=+-
  Subtract2 : Sum  Inputs=+-
  Terminator{,1..4,11} (6 alike) : Terminator
  Vector Concatenate1 : Concatenate
  X_n : Outport
  Y_n : Outport  Port=2
  V_n : Outport  Port=3
  A_n : Outport  Port=4
  wires:
  Constant4/1 -> Kinematic Steering1/1
  Bus Assignment8/1 -> Bus Selector1/1
  Follower Vehicle/4 -> Terminator1/1
  V_(n-1)/1 -> Subtract/1
  Kinematic Steering1/1 -> Terminator11/1
  Bus Selector3/1 -> Subtract2/2, X_n/1  "<X>"
  alpha/1 -> Follower Stopper Controller/5(decel)
  omega1/1 -> Follower Stopper Controller/6(dx_min)
  Coefficient of Friction: Dry/1 -> Follower Vehicle/3
  Follower Vehicle/7 -> Terminator4/1
  Subtract2/1 -> Follower Stopper Controller/3(deltaX)
  Vector Concatenate1/1 -> Follower Vehicle/1
  X_(n-1)/1 -> Subtract2/1
  omega3/1 -> Follower Stopper Controller/7(dx_activate)
  Bus Selector3/3 -> A_n/1  "<xddot>"
  Bus Selector3/2 -> Y_n/1  "<Y>"
  reference velocity/1 -> Follower Stopper Controller/1(r)
  Follower Vehicle/2 -> V_n/1, Subtract/2, Follower Stopper Controller/4(vel)
  Follower Vehicle/1 -> Bus Selector3/1
  Subtract/1 -> Follower Stopper Controller/2(deltaV)
  Follower Vehicle/5 -> Terminator2/1
  Follower Stopper Controller/1(u_cmd) -> Bus Assignment8/2
  Blank Message7/1 -> Bus Assignment8/1
  Bus Selector1/1 -> Follower Vehicle/2  "<X>"
  Kinematic Steering1/3 -> Vector Concatenate1/2
  Kinematic Steering1/2 -> Vector Concatenate1/1
  reference angle/1 -> Bus Assignment8/3
  Follower Vehicle/6 -> Terminator3/1
  Follower Vehicle/3 -> Terminator/1

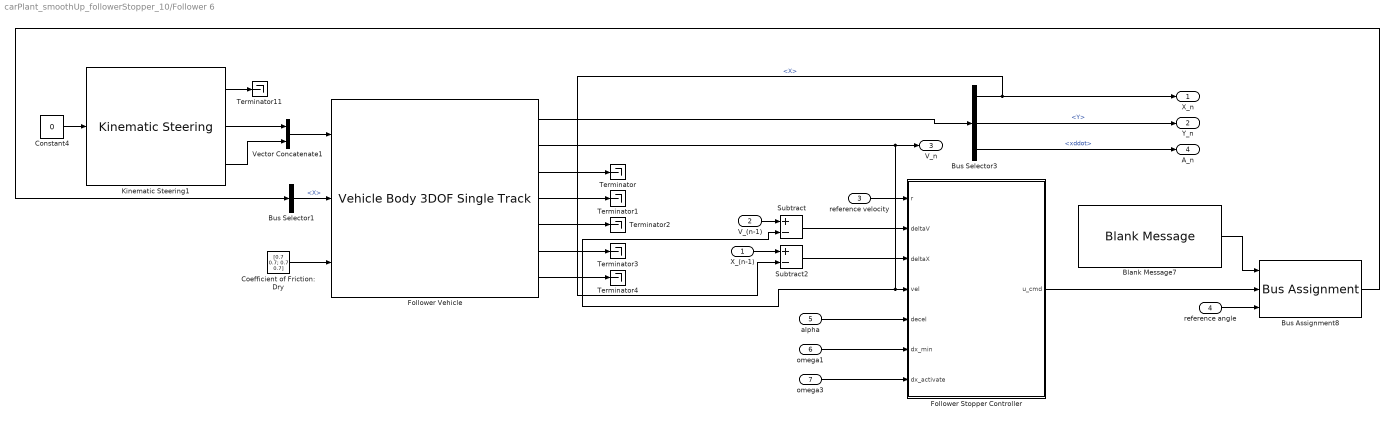
== system carPlant_smoothUp_followerStopper_10/Follower 6 ==
  X_(n-1) : Inport
  V_(n-1) : Inport  Port=2
  reference velocity : Inport  Port=3
  reference angle : Inport  Port=4
  alpha : Inport  Port=5
  omega1 : Inport  Port=6
  omega3 : Inport  Port=7
  Blank Message7 : robotlib/Blank Message  messageClass=Message  entityType=geometry_msgs/Twist  messageType=geometry_msgs/Twist  SampleTime=inf
      settings: SourceProductBaseCode=RO
  Bus Assignment8 : BusAssignment  AssignedSignals=Linear.X,Angular.Z
  Bus Selector1 : BusSelector  OutputSignals=Linear.X
  Bus Selector3 : BusSelector  OutputSignals=InertFrm.Geom.Disp.X,InertFrm.Geom.Disp.Y,BdyFrm.Cg.Acc.xddot
  Coefficient of Friction: Dry : Constant  Value=[0.7 0.7; 0.7 0.7]
  Constant4 : Constant  Value=0
  Follower Stopper Controller : Subsystem
  Follower Vehicle : autolibshared/Vehicle Body 3DOF Single Track  trackMode=Dual  inputMode=External longitudinal velocity  frontSteerMode=on  rearSteerMode=off  windMode=off  muMode=on  extFMode=off  extMMode=off  aMode=2  NF=2  NR=2  m=2000  a=1.4  b=1.6  h=0.35  X_o=15  xdot_o=0  CalphaMode=off  sigmaMode=on  d=0  w=[1.4,1.4]  Cy_f=12e3  Cy_r=11e3  sigma_f=.1  sigma_r=.1  alpha_f_brk=[-.1 .1]  Cy_f_data=[-9e3 9e3]  alpha_r_brk=[-.1 .1]  Cy_r_data=[-9e3 9e3]  Y_o=0  ydot_o=0  Izz=4000  psi_o=0  r_o=0  Af=2  Cd=.3  Cl=.1  Cpm=.1  beta_w=[0:0.01:0.3]  Cs=[0:0.03:0.9]  Cym=[0:0.01:0.3]  Pabs=101325  Tair=273  g=9.81  mu=1  xdot_tol=.01  Fznom=5000  Fxtire_sat=7e4  Fytire_sat=7e4  longOff=0  latOff=0  vertOff=0
      settings: SourceProductName=Powertrain Blockset  SourceProductBaseCode=PW
  Kinematic Steering1 : vehdynlibsteering/Kinematic Steering  StrgType=Rack and pinion  StrgRatioType=Constant  Loc=Front  NrmlFctr=0.01  TrckWdth=1  WhlBase=1.524  Db=0  StrgRng=1.25*pi  StrgAngBpts="[-6.2832   -5.0265   -3.7699   -2.5133   -1.2566         0    1.2566    2.5133    3.7699    5.0265    6.2832]"  StrgRatioTbl=|  StrgRatio=100  StrgArmLngth=0.1  RckCsLngth=0.5  TieRodLngth=0.248  D=0.2  PnnRadius=0.0057  PnnRadiusTbl="[0.0055    0.0055    0.0056    0.0057    0.0058    0.0057    0.0057    0.0057    0.0056    0.0055    0.0055]"  RodLngth=0.1  ParaArmLngth=0.9  aMode=2
      | [13.5000   13.3750   13.2500   13.1250   13.0000   13.0000   13.0000   13.1250   13.2500   13.3750   13.5000
      | ]
      settings: SourceProductName=Vehicle Dynamics Blockset
  Subtract : Sum  Inputs=+-
  Subtract2 : Sum  Inputs=+-
  Terminator{,1..4,11} (6 alike) : Terminator
  Vector Concatenate1 : Concatenate
  X_n : Outport
  Y_n : Outport  Port=2
  V_n : Outport  Port=3
  A_n : Outport  Port=4
  wires:
  Follower Vehicle/3 -> Terminator/1
  Follower Vehicle/6 -> Terminator3/1
  reference angle/1 -> Bus Assignment8/3
  Kinematic Steering1/2 -> Vector Concatenate1/1
  Kinematic Steering1/3 -> Vector Concatenate1/2
  Bus Selector1/1 -> Follower Vehicle/2  "<X>"
  Blank Message7/1 -> Bus Assignment8/1
  Follower Stopper Controller/1(u_cmd) -> Bus Assignment8/2
  Follower Vehicle/5 -> Terminator2/1
  Subtract/1 -> Follower Stopper Controller/2(deltaV)
  Follower Vehicle/1 -> Bus Selector3/1
  Follower Vehicle/2 -> Follower Stopper Controller/4(vel), Subtract/2, V_n/1
  reference velocity/1 -> Follower Stopper Controller/1(r)
  Bus Selector3/2 -> Y_n/1  "<Y>"
  Bus Selector3/3 -> A_n/1  "<xddot>"
  omega3/1 -> Follower Stopper Controller/7(dx_activate)
  X_(n-1)/1 -> Subtract2/1
  Vector Concatenate1/1 -> Follower Vehicle/1
  Subtract2/1 -> Follower Stopper Controller/3(deltaX)
  Follower Vehicle/7 -> Terminator4/1
  Coefficient of Friction: Dry/1 -> Follower Vehicle/3
  omega1/1 -> Follower Stopper Controller/6(dx_min)
  alpha/1 -> Follower Stopper Controller/5(decel)
  Bus Selector3/1 -> X_n/1, Subtract2/2  "<X>"
  Kinematic Steering1/1 -> Terminator11/1
  V_(n-1)/1 -> Subtract/1
  Follower Vehicle/4 -> Terminator1/1
  Bus Assignment8/1 -> Bus Selector1/1
  Constant4/1 -> Kinematic Steering1/1

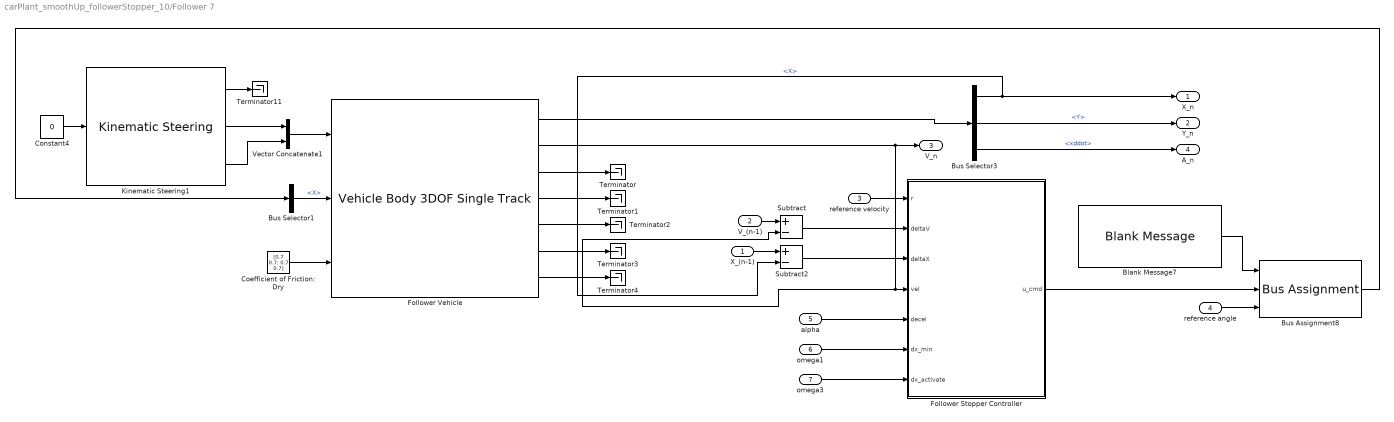
== system carPlant_smoothUp_followerStopper_10/Follower 7 ==
  X_(n-1) : Inport
  V_(n-1) : Inport  Port=2
  reference velocity : Inport  Port=3
  reference angle : Inport  Port=4
  alpha : Inport  Port=5
  omega1 : Inport  Port=6
  omega3 : Inport  Port=7
  Blank Message7 : robotlib/Blank Message  messageClass=Message  entityType=geometry_msgs/Twist  messageType=geometry_msgs/Twist  SampleTime=inf
      settings: SourceProductBaseCode=RO
  Bus Assignment8 : BusAssignment  AssignedSignals=Linear.X,Angular.Z
  Bus Selector1 : BusSelector  OutputSignals=Linear.X
  Bus Selector3 : BusSelector  OutputSignals=InertFrm.Geom.Disp.X,InertFrm.Geom.Disp.Y,BdyFrm.Cg.Acc.xddot
  Coefficient of Friction: Dry : Constant  Value=[0.7 0.7; 0.7 0.7]
  Constant4 : Constant  Value=0
  Follower Stopper Controller : Subsystem
  Follower Vehicle : autolibshared/Vehicle Body 3DOF Single Track  trackMode=Dual  inputMode=External longitudinal velocity  frontSteerMode=on  rearSteerMode=off  windMode=off  muMode=on  extFMode=off  extMMode=off  aMode=2  NF=2  NR=2  m=2000  a=1.4  b=1.6  h=0.35  X_o=10  xdot_o=0  CalphaMode=off  sigmaMode=on  d=0  w=[1.4,1.4]  Cy_f=12e3  Cy_r=11e3  sigma_f=.1  sigma_r=.1  alpha_f_brk=[-.1 .1]  Cy_f_data=[-9e3 9e3]  alpha_r_brk=[-.1 .1]  Cy_r_data=[-9e3 9e3]  Y_o=0  ydot_o=0  Izz=4000  psi_o=0  r_o=0  Af=2  Cd=.3  Cl=.1  Cpm=.1  beta_w=[0:0.01:0.3]  Cs=[0:0.03:0.9]  Cym=[0:0.01:0.3]  Pabs=101325  Tair=273  g=9.81  mu=1  xdot_tol=.01  Fznom=5000  Fxtire_sat=7e4  Fytire_sat=7e4  longOff=0  latOff=0  vertOff=0
      settings: SourceProductName=Powertrain Blockset  SourceProductBaseCode=PW
  Kinematic Steering1 : vehdynlibsteering/Kinematic Steering  StrgType=Rack and pinion  StrgRatioType=Constant  Loc=Front  NrmlFctr=0.01  TrckWdth=1  WhlBase=1.524  Db=0  StrgRng=1.25*pi  StrgAngBpts="[-6.2832   -5.0265   -3.7699   -2.5133   -1.2566         0    1.2566    2.5133    3.7699    5.0265    6.2832]"  StrgRatioTbl=|  StrgRatio=100  StrgArmLngth=0.1  RckCsLngth=0.5  TieRodLngth=0.248  D=0.2  PnnRadius=0.0057  PnnRadiusTbl="[0.0055    0.0055    0.0056    0.0057    0.0058    0.0057    0.0057    0.0057    0.0056    0.0055    0.0055]"  RodLngth=0.1  ParaArmLngth=0.9  aMode=2
      | [13.5000   13.3750   13.2500   13.1250   13.0000   13.0000   13.0000   13.1250   13.2500   13.3750   13.5000
      | ]
      settings: SourceProductName=Vehicle Dynamics Blockset
  Subtract : Sum  Inputs=+-
  Subtract2 : Sum  Inputs=+-
  Terminator{,1..4,11} (6 alike) : Terminator
  Vector Concatenate1 : Concatenate
  X_n : Outport
  Y_n : Outport  Port=2
  V_n : Outport  Port=3
  A_n : Outport  Port=4
  wires:
  Constant4/1 -> Kinematic Steering1/1
  Bus Assignment8/1 -> Bus Selector1/1
  Follower Vehicle/4 -> Terminator1/1
  V_(n-1)/1 -> Subtract/1
  Kinematic Steering1/1 -> Terminator11/1
  Bus Selector3/1 -> Subtract2/2, X_n/1  "<X>"
  alpha/1 -> Follower Stopper Controller/5(decel)
  omega1/1 -> Follower Stopper Controller/6(dx_min)
  Coefficient of Friction: Dry/1 -> Follower Vehicle/3
  Follower Vehicle/7 -> Terminator4/1
  Subtract2/1 -> Follower Stopper Controller/3(deltaX)
  Vector Concatenate1/1 -> Follower Vehicle/1
  X_(n-1)/1 -> Subtract2/1
  omega3/1 -> Follower Stopper Controller/7(dx_activate)
  Bus Selector3/3 -> A_n/1  "<xddot>"
  Bus Selector3/2 -> Y_n/1  "<Y>"
  reference velocity/1 -> Follower Stopper Controller/1(r)
  Follower Vehicle/2 -> V_n/1, Subtract/2, Follower Stopper Controller/4(vel)
  Follower Vehicle/1 -> Bus Selector3/1
  Subtract/1 -> Follower Stopper Controller/2(deltaV)
  Follower Vehicle/5 -> Terminator2/1
  Follower Stopper Controller/1(u_cmd) -> Bus Assignment8/2
  Blank Message7/1 -> Bus Assignment8/1
  Bus Selector1/1 -> Follower Vehicle/2  "<X>"
  Kinematic Steering1/3 -> Vector Concatenate1/2
  Kinematic Steering1/2 -> Vector Concatenate1/1
  reference angle/1 -> Bus Assignment8/3
  Follower Vehicle/6 -> Terminator3/1
  Follower Vehicle/3 -> Terminator/1

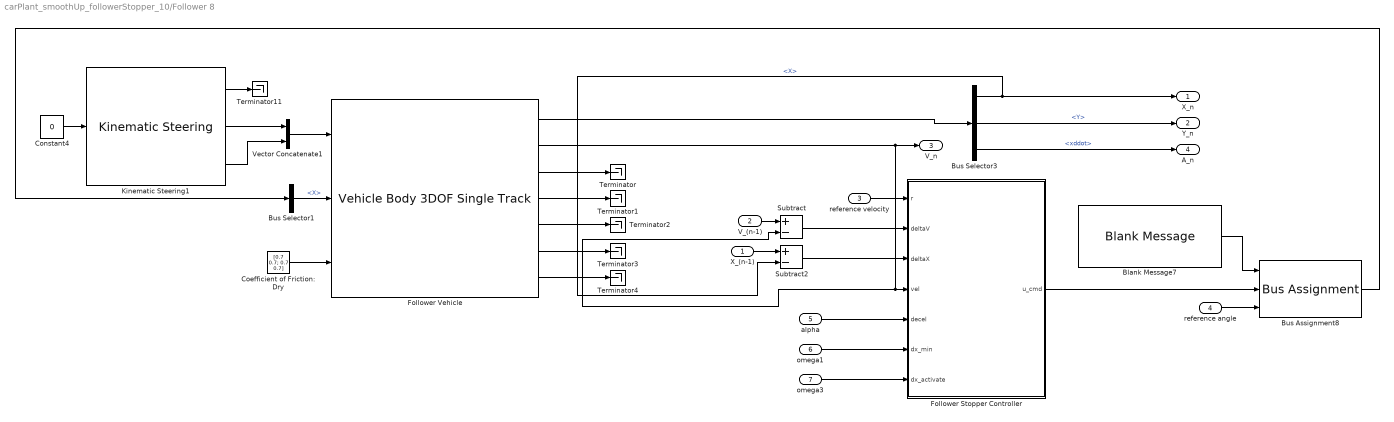
== system carPlant_smoothUp_followerStopper_10/Follower 8 ==
  X_(n-1) : Inport
  V_(n-1) : Inport  Port=2
  reference velocity : Inport  Port=3
  reference angle : Inport  Port=4
  alpha : Inport  Port=5
  omega1 : Inport  Port=6
  omega3 : Inport  Port=7
  Blank Message7 : robotlib/Blank Message  messageClass=Message  entityType=geometry_msgs/Twist  messageType=geometry_msgs/Twist  SampleTime=inf
      settings: SourceProductBaseCode=RO
  Bus Assignment8 : BusAssignment  AssignedSignals=Linear.X,Angular.Z
  Bus Selector1 : BusSelector  OutputSignals=Linear.X
  Bus Selector3 : BusSelector  OutputSignals=InertFrm.Geom.Disp.X,InertFrm.Geom.Disp.Y,BdyFrm.Cg.Acc.xddot
  Coefficient of Friction: Dry : Constant  Value=[0.7 0.7; 0.7 0.7]
  Constant4 : Constant  Value=0
  Follower Stopper Controller : Subsystem
  Follower Vehicle : autolibshared/Vehicle Body 3DOF Single Track  trackMode=Dual  inputMode=External longitudinal velocity  frontSteerMode=on  rearSteerMode=off  windMode=off  muMode=on  extFMode=off  extMMode=off  aMode=2  NF=2  NR=2  m=2000  a=1.4  b=1.6  h=0.35  X_o=5  xdot_o=0  CalphaMode=off  sigmaMode=on  d=0  w=[1.4,1.4]  Cy_f=12e3  Cy_r=11e3  sigma_f=.1  sigma_r=.1  alpha_f_brk=[-.1 .1]  Cy_f_data=[-9e3 9e3]  alpha_r_brk=[-.1 .1]  Cy_r_data=[-9e3 9e3]  Y_o=0  ydot_o=0  Izz=4000  psi_o=0  r_o=0  Af=2  Cd=.3  Cl=.1  Cpm=.1  beta_w=[0:0.01:0.3]  Cs=[0:0.03:0.9]  Cym=[0:0.01:0.3]  Pabs=101325  Tair=273  g=9.81  mu=1  xdot_tol=.01  Fznom=5000  Fxtire_sat=7e4  Fytire_sat=7e4  longOff=0  latOff=0  vertOff=0
      settings: SourceProductName=Powertrain Blockset  SourceProductBaseCode=PW
  Kinematic Steering1 : vehdynlibsteering/Kinematic Steering  StrgType=Rack and pinion  StrgRatioType=Constant  Loc=Front  NrmlFctr=0.01  TrckWdth=1  WhlBase=1.524  Db=0  StrgRng=1.25*pi  StrgAngBpts="[-6.2832   -5.0265   -3.7699   -2.5133   -1.2566         0    1.2566    2.5133    3.7699    5.0265    6.2832]"  StrgRatioTbl=|  StrgRatio=100  StrgArmLngth=0.1  RckCsLngth=0.5  TieRodLngth=0.248  D=0.2  PnnRadius=0.0057  PnnRadiusTbl="[0.0055    0.0055    0.0056    0.0057    0.0058    0.0057    0.0057    0.0057    0.0056    0.0055    0.0055]"  RodLngth=0.1  ParaArmLngth=0.9  aMode=2
      | [13.5000   13.3750   13.2500   13.1250   13.0000   13.0000   13.0000   13.1250   13.2500   13.3750   13.5000
      | ]
      settings: SourceProductName=Vehicle Dynamics Blockset
  Subtract : Sum  Inputs=+-
  Subtract2 : Sum  Inputs=+-
  Terminator{,1..4,11} (6 alike) : Terminator
  Vector Concatenate1 : Concatenate
  X_n : Outport
  Y_n : Outport  Port=2
  V_n : Outport  Port=3
  A_n : Outport  Port=4
  wires:
  Follower Vehicle/3 -> Terminator/1
  Follower Vehicle/6 -> Terminator3/1
  reference angle/1 -> Bus Assignment8/3
  Kinematic Steering1/2 -> Vector Concatenate1/1
  Kinematic Steering1/3 -> Vector Concatenate1/2
  Bus Selector1/1 -> Follower Vehicle/2  "<X>"
  Blank Message7/1 -> Bus Assignment8/1
  Follower Stopper Controller/1(u_cmd) -> Bus Assignment8/2
  Follower Vehicle/5 -> Terminator2/1
  Subtract/1 -> Follower Stopper Controller/2(deltaV)
  Follower Vehicle/1 -> Bus Selector3/1
  Follower Vehicle/2 -> Follower Stopper Controller/4(vel), Subtract/2, V_n/1
  reference velocity/1 -> Follower Stopper Controller/1(r)
  Bus Selector3/2 -> Y_n/1  "<Y>"
  Bus Selector3/3 -> A_n/1  "<xddot>"
  omega3/1 -> Follower Stopper Controller/7(dx_activate)
  X_(n-1)/1 -> Subtract2/1
  Vector Concatenate1/1 -> Follower Vehicle/1
  Subtract2/1 -> Follower Stopper Controller/3(deltaX)
  Follower Vehicle/7 -> Terminator4/1
  Coefficient of Friction: Dry/1 -> Follower Vehicle/3
  omega1/1 -> Follower Stopper Controller/6(dx_min)
  alpha/1 -> Follower Stopper Controller/5(decel)
  Bus Selector3/1 -> X_n/1, Subtract2/2  "<X>"
  Kinematic Steering1/1 -> Terminator11/1
  V_(n-1)/1 -> Subtract/1
  Follower Vehicle/4 -> Terminator1/1
  Bus Assignment8/1 -> Bus Selector1/1
  Constant4/1 -> Kinematic Steering1/1

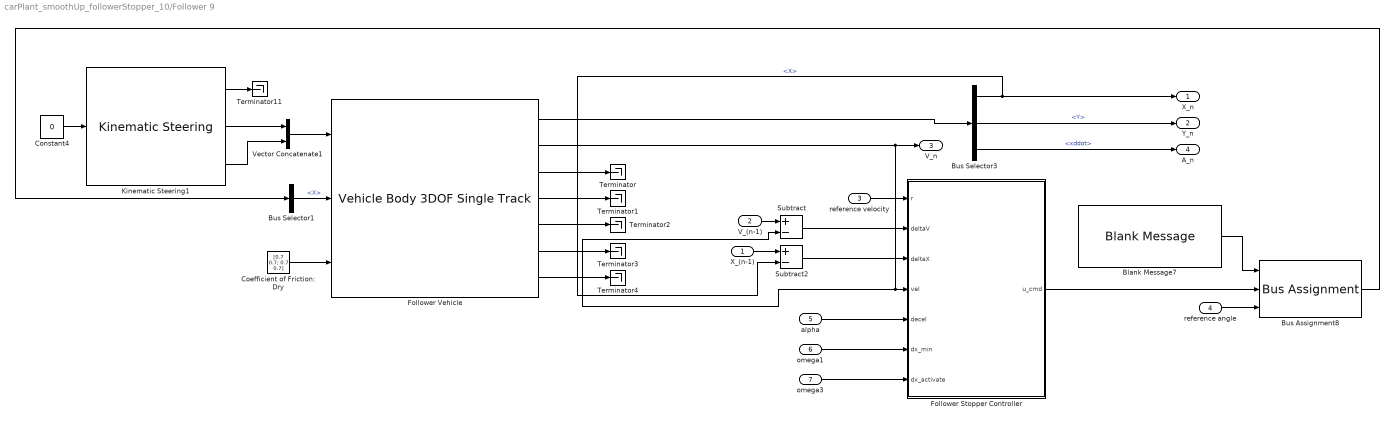
== system carPlant_smoothUp_followerStopper_10/Follower 9 ==
  X_(n-1) : Inport
  V_(n-1) : Inport  Port=2
  reference velocity : Inport  Port=3
  reference angle : Inport  Port=4
  alpha : Inport  Port=5
  omega1 : Inport  Port=6
  omega3 : Inport  Port=7
  Blank Message7 : robotlib/Blank Message  messageClass=Message  entityType=geometry_msgs/Twist  messageType=geometry_msgs/Twist  SampleTime=inf
      settings: SourceProductBaseCode=RO
  Bus Assignment8 : BusAssignment  AssignedSignals=Linear.X,Angular.Z
  Bus Selector1 : BusSelector  OutputSignals=Linear.X
  Bus Selector3 : BusSelector  OutputSignals=InertFrm.Geom.Disp.X,InertFrm.Geom.Disp.Y,BdyFrm.Cg.Acc.xddot
  Coefficient of Friction: Dry : Constant  Value=[0.7 0.7; 0.7 0.7]
  Constant4 : Constant  Value=0
  Follower Stopper Controller : Subsystem
  Follower Vehicle : autolibshared/Vehicle Body 3DOF Single Track  trackMode=Dual  inputMode=External longitudinal velocity  frontSteerMode=on  rearSteerMode=off  windMode=off  muMode=on  extFMode=off  extMMode=off  aMode=2  NF=2  NR=2  m=2000  a=1.4  b=1.6  h=0.35  X_o=0  xdot_o=0  CalphaMode=off  sigmaMode=on  d=0  w=[1.4,1.4]  Cy_f=12e3  Cy_r=11e3  sigma_f=.1  sigma_r=.1  alpha_f_brk=[-.1 .1]  Cy_f_data=[-9e3 9e3]  alpha_r_brk=[-.1 .1]  Cy_r_data=[-9e3 9e3]  Y_o=0  ydot_o=0  Izz=4000  psi_o=0  r_o=0  Af=2  Cd=.3  Cl=.1  Cpm=.1  beta_w=[0:0.01:0.3]  Cs=[0:0.03:0.9]  Cym=[0:0.01:0.3]  Pabs=101325  Tair=273  g=9.81  mu=1  xdot_tol=.01  Fznom=5000  Fxtire_sat=7e4  Fytire_sat=7e4  longOff=0  latOff=0  vertOff=0
      settings: SourceProductName=Powertrain Blockset  SourceProductBaseCode=PW
  Kinematic Steering1 : vehdynlibsteering/Kinematic Steering  StrgType=Rack and pinion  StrgRatioType=Constant  Loc=Front  NrmlFctr=0.01  TrckWdth=1  WhlBase=1.524  Db=0  StrgRng=1.25*pi  StrgAngBpts="[-6.2832   -5.0265   -3.7699   -2.5133   -1.2566         0    1.2566    2.5133    3.7699    5.0265    6.2832]"  StrgRatioTbl=|  StrgRatio=100  StrgArmLngth=0.1  RckCsLngth=0.5  TieRodLngth=0.248  D=0.2  PnnRadius=0.0057  PnnRadiusTbl="[0.0055    0.0055    0.0056    0.0057    0.0058    0.0057    0.0057    0.0057    0.0056    0.0055    0.0055]"  RodLngth=0.1  ParaArmLngth=0.9  aMode=2
      | [13.5000   13.3750   13.2500   13.1250   13.0000   13.0000   13.0000   13.1250   13.2500   13.3750   13.5000
      | ]
      settings: SourceProductName=Vehicle Dynamics Blockset
  Subtract : Sum  Inputs=+-
  Subtract2 : Sum  Inputs=+-
  Terminator{,1..4,11} (6 alike) : Terminator
  Vector Concatenate1 : Concatenate
  X_n : Outport
  Y_n : Outport  Port=2
  V_n : Outport  Port=3
  A_n : Outport  Port=4
  wires:
  Constant4/1 -> Kinematic Steering1/1
  Bus Assignment8/1 -> Bus Selector1/1
  Follower Vehicle/4 -> Terminator1/1
  V_(n-1)/1 -> Subtract/1
  Kinematic Steering1/1 -> Terminator11/1
  Bus Selector3/1 -> Subtract2/2, X_n/1  "<X>"
  alpha/1 -> Follower Stopper Controller/5(decel)
  omega1/1 -> Follower Stopper Controller/6(dx_min)
  Coefficient of Friction: Dry/1 -> Follower Vehicle/3
  Follower Vehicle/7 -> Terminator4/1
  Subtract2/1 -> Follower Stopper Controller/3(deltaX)
  Vector Concatenate1/1 -> Follower Vehicle/1
  X_(n-1)/1 -> Subtract2/1
  omega3/1 -> Follower Stopper Controller/7(dx_activate)
  Bus Selector3/3 -> A_n/1  "<xddot>"
  Bus Selector3/2 -> Y_n/1  "<Y>"
  reference velocity/1 -> Follower Stopper Controller/1(r)
  Follower Vehicle/2 -> V_n/1, Subtract/2, Follower Stopper Controller/4(vel)
  Follower Vehicle/1 -> Bus Selector3/1
  Subtract/1 -> Follower Stopper Controller/2(deltaV)
  Follower Vehicle/5 -> Terminator2/1
  Follower Stopper Controller/1(u_cmd) -> Bus Assignment8/2
  Blank Message7/1 -> Bus Assignment8/1
  Bus Selector1/1 -> Follower Vehicle/2  "<X>"
  Kinematic Steering1/3 -> Vector Concatenate1/2
  Kinematic Steering1/2 -> Vector Concatenate1/1
  reference angle/1 -> Bus Assignment8/3
  Follower Vehicle/6 -> Terminator3/1
  Follower Vehicle/3 -> Terminator/1

== system carPlant_smoothUp_followerStopper_10/Parameters ==
  note: \alpha_{1,2,3}
  note: \omega_1
  note: \omega_3
  Get Parameter1 : robotlib/Get Parameter  ParameterSource=Specify your own  ParameterName=/dx_min  ParameterType=double  ParameterMaxArrayLength=16  ParameterInitialValue=4.5  SampleTime=-1  ShowErrorCodeOutput=off  ModelName=carPlant_smoothUp_followerStopper_10  BlockId=ParamGet_carPlant_smoothUp_followerStopper_10_57
      settings: SourceProductName=Robotics System Toolbox  SourceProductBaseCode=RO
  Get Parameter2 : robotlib/Get Parameter  ParameterSource=Specify your own  ParameterName=/dx_activate  ParameterType=double  ParameterMaxArrayLength=16  ParameterInitialValue=6.0  SampleTime=-1  ShowErrorCodeOutput=off  ModelName=carPlant_smoothUp_followerStopper_10  BlockId=ParamGet_carPlant_smoothUp_followerStopper_10_58
      settings: SourceProductName=Robotics System Toolbox  SourceProductBaseCode=RO
  decel : Constant  Value=[1.5 1.0 0.5]  OutDataTypeStr=double  SampleTime=-1
  alpha : Outport
  omega_1 : Outport  Port=2
  omega_3 : Outport  Port=3
  wires:
  decel/1 -> alpha/1
  Get Parameter1/1 -> omega_1/1
  Get Parameter2/1 -> omega_3/1

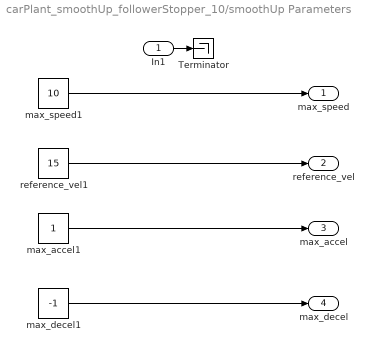
== system carPlant_smoothUp_followerStopper_10/smoothUp Parameters ==
  In1 : Inport
  Terminator : Terminator
  max_accel1 : Constant
  max_decel1 : Constant  Value=-1
  max_speed1 : Constant  Value=10
  reference_vel1 : Constant  Value=15
  max_speed : Outport  Tag=max_speed
  reference_vel : Outport  Port=2
  max_accel : Outport  Port=3
  max_decel : Outport  Port=4
  wires:
  In1/1 -> Terminator/1
  max_speed1/1 -> max_speed/1
  reference_vel1/1 -> reference_vel/1
  max_accel1/1 -> max_accel/1
  max_decel1/1 -> max_decel/1

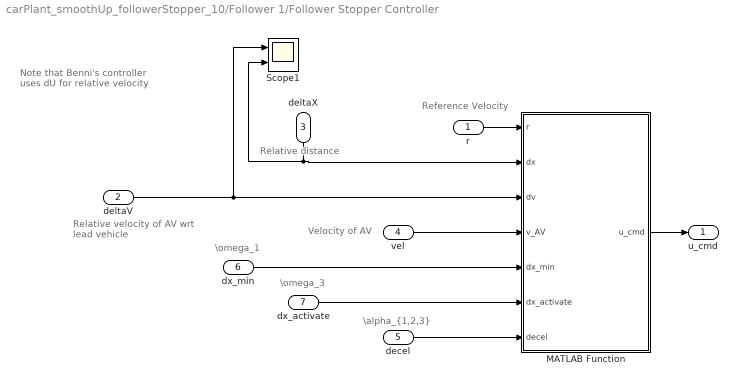
== system carPlant_smoothUp_followerStopper_10/Follower 1/Follower Stopper Controller ==
  note: \alpha_{1,2,3}
  note: \omega_3
  note: \omega_1
  note: Relative distance
  note: Reference Velocity
  note: Velocity of AV
  note: Relative velocity of
      | AV wrt lead vehicle
  note: Note that Benni's
      | controller uses dU
      | for relative
      | velocity
  r : Inport
  deltaV : Inport  Port=2
  deltaX : Inport  Port=3
  vel : Inport  Port=4
  decel : Inport  Port=5
  dx_min : Inport  Port=6
  dx_activate : Inport  Port=7
  MATLAB Function : MATLAB Function  TreatAsAtomicUnit=on
  Scope1 : Scope  NumInputPorts=2
  u_cmd : Outport
  wires:
  r/1 -> MATLAB Function/1(r)
  dx_activate/1 -> MATLAB Function/6(dx_activate)
  decel/1 -> MATLAB Function/7(decel)
  dx_min/1 -> MATLAB Function/5(dx_min)
  vel/1 -> MATLAB Function/4(v_AV)
  MATLAB Function/1(u_cmd) -> u_cmd/1
  deltaV/1 -> Scope1/1, MATLAB Function/3(dv)
  deltaX/1 -> Scope1/2, MATLAB Function/2(dx)

== system carPlant_smoothUp_followerStopper_10/Follower 2/Follower Stopper Controller ==
  note: Note that Benni's
      | controller uses dU
      | for relative
      | velocity
  note: Relative velocity of
      | AV wrt lead vehicle
  note: Velocity of AV
  note: Reference Velocity
  note: Relative distance
  note: \omega_1
  note: \omega_3
  note: \alpha_{1,2,3}
  r : Inport
  deltaV : Inport  Port=2
  deltaX : Inport  Port=3
  vel : Inport  Port=4
  decel : Inport  Port=5
  dx_min : Inport  Port=6
  dx_activate : Inport  Port=7
  MATLAB Function : MATLAB Function  TreatAsAtomicUnit=on
  Scope1 : Scope  NumInputPorts=2
  u_cmd : Outport
  wires:
  deltaX/1 -> MATLAB Function/2(dx), Scope1/2
  deltaV/1 -> MATLAB Function/3(dv), Scope1/1
  MATLAB Function/1(u_cmd) -> u_cmd/1
  vel/1 -> MATLAB Function/4(v_AV)
  dx_min/1 -> MATLAB Function/5(dx_min)
  decel/1 -> MATLAB Function/7(decel)
  dx_activate/1 -> MATLAB Function/6(dx_activate)
  r/1 -> MATLAB Function/1(r)

== system carPlant_smoothUp_followerStopper_10/Follower 3/Follower Stopper Controller ==
  note: \alpha_{1,2,3}
  note: \omega_3
  note: \omega_1
  note: Relative distance
  note: Reference Velocity
  note: Velocity of AV
  note: Relative velocity of
      | AV wrt lead vehicle
  note: Note that Benni's
      | controller uses dU
      | for relative
      | velocity
  r : Inport
  deltaV : Inport  Port=2
  deltaX : Inport  Port=3
  vel : Inport  Port=4
  decel : Inport  Port=5
  dx_min : Inport  Port=6
  dx_activate : Inport  Port=7
  MATLAB Function : MATLAB Function  TreatAsAtomicUnit=on
  Scope1 : Scope  NumInputPorts=2
  u_cmd : Outport
  wires:
  r/1 -> MATLAB Function/1(r)
  dx_activate/1 -> MATLAB Function/6(dx_activate)
  decel/1 -> MATLAB Function/7(decel)
  dx_min/1 -> MATLAB Function/5(dx_min)
  vel/1 -> MATLAB Function/4(v_AV)
  MATLAB Function/1(u_cmd) -> u_cmd/1
  deltaV/1 -> Scope1/1, MATLAB Function/3(dv)
  deltaX/1 -> Scope1/2, MATLAB Function/2(dx)

== system carPlant_smoothUp_followerStopper_10/Follower 4/Follower Stopper Controller ==
  note: Note that Benni's
      | controller uses dU
      | for relative
      | velocity
  note: Relative velocity of
      | AV wrt lead vehicle
  note: Velocity of AV
  note: Reference Velocity
  note: Relative distance
  note: \omega_1
  note: \omega_3
  note: \alpha_{1,2,3}
  r : Inport
  deltaV : Inport  Port=2
  deltaX : Inport  Port=3
  vel : Inport  Port=4
  decel : Inport  Port=5
  dx_min : Inport  Port=6
  dx_activate : Inport  Port=7
  MATLAB Function : MATLAB Function  TreatAsAtomicUnit=on
  Scope1 : Scope  NumInputPorts=2
  u_cmd : Outport
  wires:
  deltaX/1 -> MATLAB Function/2(dx), Scope1/2
  deltaV/1 -> MATLAB Function/3(dv), Scope1/1
  MATLAB Function/1(u_cmd) -> u_cmd/1
  vel/1 -> MATLAB Function/4(v_AV)
  dx_min/1 -> MATLAB Function/5(dx_min)
  decel/1 -> MATLAB Function/7(decel)
  dx_activate/1 -> MATLAB Function/6(dx_activate)
  r/1 -> MATLAB Function/1(r)
